simulink model "hybrid_sm"  (R2022b)
settings: Solver=VariableStepAuto  StartTime=0.0  StopTime=T  MaxStep=MaxStep  RelTol=RelTol
values from neighbouring files (symbols this model uses):
  J = 20    [initialization.m]
  parameters = [1,1,1;1,1,1;1,1,1]    [initialization.m]
  T = 10    [initialization.m]
libraries: HyEQ_Library x3
settings Model: Creator=tom  LastModifiedBy=tom

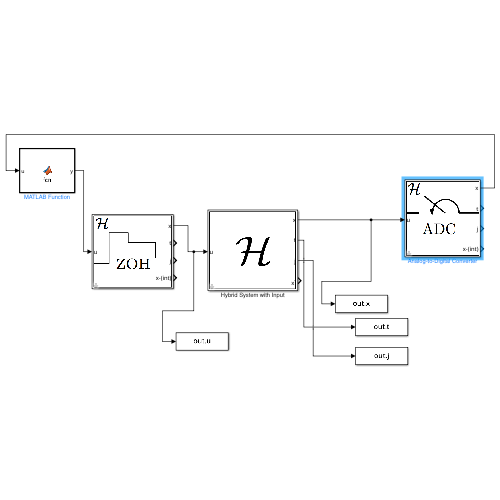
[thumbnail: Simulink's stored preview of the top-level diagram]
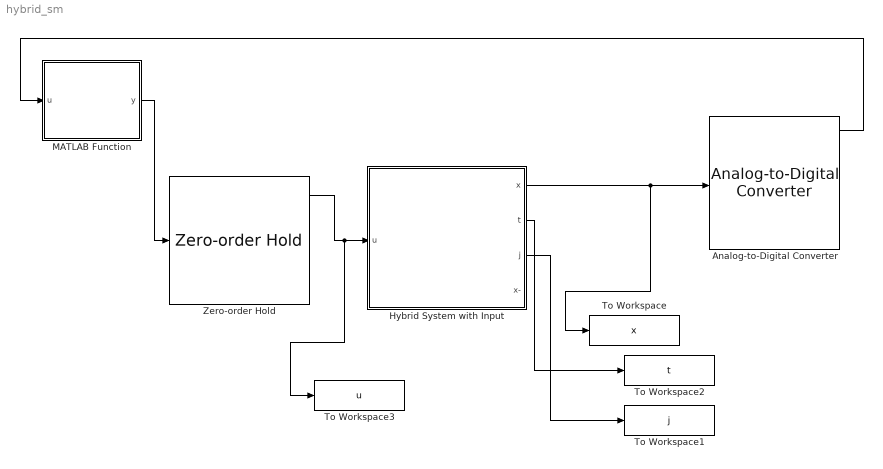
== system hybrid_sm ==
  Analog-to-Digital Converter : HyEQ_Library/Cyber Physical Systems/Analog-to-Digital Converter  sample_time=1  u0=[0]  tau0=tau_0  T=T  J=J
      settings: SourceProductName=Hybrid Equations Toolbox
  Hybrid System with Input : Subsystem  LoadFcn=set_param(gcb,'LinkStatus','none')  mask(Hybrid System with Inputs){x0=0, input_dim=2, parameters=parameters, T=T, J=J, rule=Jump}
      mask prompts: x0 "Initial Condition (column vector)"; input_dim "Input Dimension (positive integer)"; T "Flow Horizon (nonnegative real)"; J "Jump Horizon (nonnegative integer)"; rule "Flow/Jump Priorty Rule"
      mask help:
      | To modify (f, g, C, D) for this block, "Look inside" the block mask by either clicking the down arrow in the lower-left corner or selecting "Mask" > "Look Under Mask" from the context menu.
      |
      | For instructions how to use this block, see the
      mask init:
      | state_dim = numel(x0);
      settings: CopyFcn=|
      | set_param(gcb,'LinkStatus','none'),
      | set_param(gcs, 'MaxStep', 'MaxStep', 'RelTol', 'RelTol','StopTime', 'T')
      mask Help:
      | To modify (f, g, C, D) for this block, "Look inside" the block mask by either clicking the down arrow in the lower-left corner or selecting "Mask" > "Look Under Mask" from the context menu.
      | 
      | The value given in the 'parameters' field is passed as the last input argument for f, g, C, and D. Any MATLAB object can be used, but we recommend using a struct. For example, in the initialization script, a parameters struct can be defined as followed.
      |   parameters = struct();
      |   parameters.A = eye(2);
      |   parameters.B = [1; 0];
      | 
      | The output "x-" is the state output delayed by one integration step. Use this output to break algebraic loops.
      mask TypeOptions x0: Integrator System/x0
      mask TypeOptions T: Integrator System/T
      mask TypeOptions J: Integrator System/J
      mask TypeOptions rule: Jump | Flow | Random
      mask DialogControl Control2 Prompt: Introduction to the HyEQ Simulink-based Library
      mask DialogControl Control2 Callback: hybrid.internal.openHelp('Help_SimulinkLibrary')
      mask DialogControl Container3 Prompt: System Configuration
      mask DialogControl Container2 Prompt: Solver Options
      mask Display:
      | image('Hcal.jpg')
      | port_label('output', 1, 'x')
      | port_label('output', 2, 't')
      | port_label('output', 3, 'j')
      | port_label('output', 4, 'x^-','texmode', 'on')
      | port_label('input', 1, 'u')
  MATLAB Function : MATLAB Function  TreatAsAtomicUnit=on
  To Workspace : ToWorkspace  VariableName=x  SaveFormat=Timeseries  SampleTime=-1
  To Workspace1 : ToWorkspace  VariableName=j  SaveFormat=Timeseries  SampleTime=-1
  To Workspace2 : ToWorkspace  VariableName=t  SaveFormat=Timeseries  SampleTime=-1
  To Workspace3 : ToWorkspace  VariableName=u  SaveFormat=Timeseries  SampleTime=-1
  Zero-order Hold : HyEQ_Library/Cyber Physical Systems/Zero-order Hold  sample_time=1  u0=[0]  tau0=tau_0  T=T  J=J
      settings: SourceProductName=Hybrid Equations Toolbox
  wires:
  Zero-order Hold/1 -> To Workspace3/1, Hybrid System with Input/1(u)
  Hybrid System with Input/1(x) -> To Workspace/1, Analog-to-Digital Converter/1
  Analog-to-Digital Converter/1 -> MATLAB Function/1(u)
  MATLAB Function/1(y) -> Zero-order Hold/1
  Hybrid System with Input/3(j) -> To Workspace1/1
  Hybrid System with Input/2(t) -> To Workspace2/1

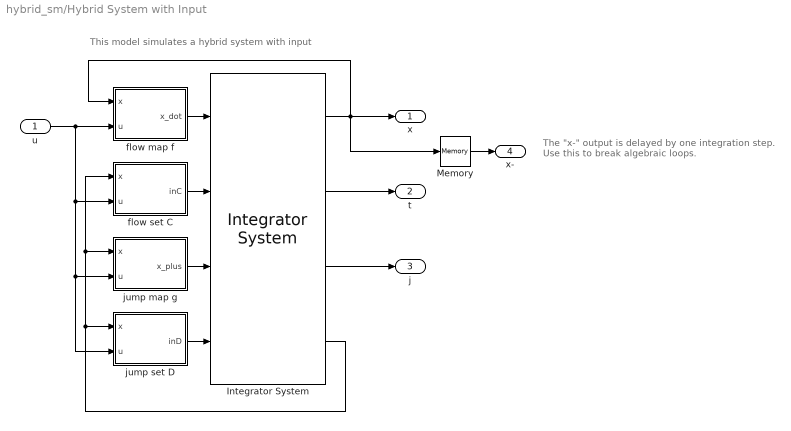
== system hybrid_sm/Hybrid System with Input ==
  note: This model simulates a hybrid system with input
  note: The "x-" output is delayed by one integration step. Use this to break algebraic loops.
  u : Inport  PortDimensions=input_dim
  Integrator System : HyEQ_Library/Other/Integrator System  Priority=2  T=T  J=J  x0=x0  rule=rule
      settings: SourceProductName=Hybrid Equations Toolbox
  Memory : Memory  InitialCondition=x0
  flow map f : MATLAB Function  TreatAsAtomicUnit=on
  flow set C : MATLAB Function  TreatAsAtomicUnit=on
  jump map g : MATLAB Function  TreatAsAtomicUnit=on
  jump set D : MATLAB Function  TreatAsAtomicUnit=on
  x : Outport  PortDimensions=state_dim
  t : Outport  Port=2  PortDimensions=1
  j : Outport  Port=3  PortDimensions=1
  x- : Outport  Port=4  PortDimensions=state_dim
  wires:
  Memory/1 -> x-/1
  jump map g/1(x_plus) -> Integrator System/3
  jump set D/1(inD) -> Integrator System/4
  u/1 -> jump set D/2(u), jump map g/2(u), flow set C/2(u), flow map f/2(u)
  Integrator System/3 -> j/1
  Integrator System/2 -> t/1
  flow set C/1(inC) -> Integrator System/2
  Integrator System/1 -> x/1, flow map f/1(x), Memory/1
  Integrator System/4 -> jump map g/1(x), flow set C/1(x), jump set D/1(x)
  flow map f/1(x_dot) -> Integrator System/1

== matlab function hybrid_sm/Hybrid System with Input/flow map f ==
  data: x input size=state_dim; u input size=input_dim; x_dot output size=state_dim; parameters parameter
function x_dot = f(x, u, parameters)
   % Define flow map here.
   %x_dot = -x + u;
   %A = parameters(:,1:2);
   %B = parameters(:,3);
   A=[1];
   B=[1];
   x_dot = A*x + B*u(2);
end

== matlab function hybrid_sm/Hybrid System with Input/flow set C ==
  data: x input size=state_dim; u input size=input_dim; inC output size=1; parameters parameter
function inC = C(x, u, parameters)
   % Define flow set indictor function here.
   inC = 1;
end

== matlab function hybrid_sm/Hybrid System with Input/jump map g ==
  data: x input size=state_dim; u input size=input_dim; x_plus output size=state_dim; parameters parameter
function x_plus = g(x, u, parameters)
   % Jump map.
   x_plus = x;
end

== matlab function hybrid_sm/Hybrid System with Input/jump set D ==
  data: x input size=state_dim; u input size=input_dim; inD output size=1; parameters parameter
function inD = D(x, u, parameters)
   % Define jump set indicator function here.
   inD = false;
end

== matlab function hybrid_sm/MATLAB Function ==
  data: u input; y output
function y = fcn(u)

y = u(1);
